simulink model "test2"  (R2012b)
settings: Solver=ode45  StartTime=0.0  StopTime=10.0  RelTol=1e-3
undefined symbols (not defined in the file or in its folder): jet
libraries: visionsources x1, visionsinks x1
settings Model: Creator=hp  LastModifiedBy=hp
settings HardwareCC: TargetIntDivRoundTo=Zero  TargetEndianess=LittleEndian  TargetHWDeviceType=MATLAB Host  ProdEqTarget=off
settings RTWCC: SystemTargetFile=rsim.tlc  GenCodeOnly=on  TemplateMakefile=rsim_default_tmf  Description=Rapid Simulation Target  ProcessScript=rsim_make_rtw_hook
settings RSimTargetCC: CodeReplacementLibrary=ANSI_C  ERTMultiwordTypeDef=System defined  ERTMultiwordLength=256  IsPILTarget=off  EnableShiftOperators=on

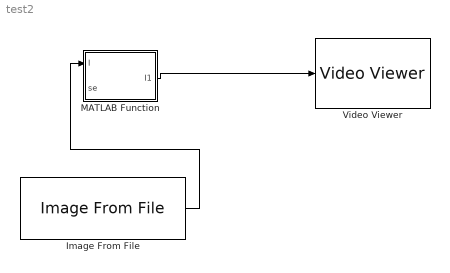
== system test2 ==
  Image From File : visionsources/Image From File  Tag=vipblks_nd  FileName=wirebond.tif  imagePorts=One multidimensional signal  Ts=inf  ImageDataType=Inherit from input image  Signed=on  WordLength=16  sdImageDataType=uint(8)  FractionLengthMode=User-defined  FractionLength=15  OutPortLabels=R|G|B
  MATLAB Function : MATLAB Function  TreatAsAtomicUnit=on
  Video Viewer : visionsinks/Video Viewer  inputType=Obsolete7b  imagePorts=One multidimensional signal  useColorMap=off  colormapValue=jet(256)  specRange=off  minInputVal=0  maxInputVal=255  FigPos=[755 749 410 300]  AxisZoom=on  trueSizedOnce=off  OpenAtMdlStart=on  DefaultConfigurationName=vipscopes.VideoViewerScopeCfg
  wires:
  Image From File/1 -> MATLAB Function/1(I)
  MATLAB Function/1(I1) -> Video Viewer/1

== matlab function test2/MATLAB Function ==
  data: I input; I1 output; se input
function I1 =dil_m(I,se)

%I = imread('text_gaps.tif');
%I(445:508,1:508)=false;
%I=true(10,10);
%figure,imshow(I);
[m,n]=size(I);
I1=false(m,n);
%se=true(3,3);
se=rflctn(se);
[sm,sn]=size(se);
p=fix(sm/2);
r=fix(sn/2);

J=false(1:m+2*p,1:n+2*r);
for i=1:m;
    for j=1:n;
        %if(i>p && i<m+p+1)
            %if(j>p && j<m+p+1)
                J(i+p,j+r)=I(i,j);
            %end 
        %end
    end
end
%figure,imshow(J);
for i=p+1:m+p;
    for j=r+1:n+r;
        q=1;
        q1=J(i-p:i+p,j-r:j+r).*se;
        if(se==1)
            if(q1==0)
                q=0;
            end
        else
            q=0;
            for si=1:2*p+1;
                for sj=1:2*r+1;
                    if(se(si,sj)==true)
                        if(q1(si,sj)==true)
                            q=1;break;
                        end
                    end
                end
                if(q==1)
                   break;
                end
            end     
        end
        if(q==0)
           I1(i-p,j-r)=false;
        else
           I1(i-p,j-r)=true;
        end
    end
end
end
